simulink model "Controller"  (R2015b)
settings: Solver=FixedStepAuto  StartTime=0.0  StopTime=10.0  FixedStep=0.1  RelTol=1e-3
undefined symbols (not defined in the file): controller_p
libraries: simulink x2
settings Model: Creator=Deepak  LastModifiedBy=Deepak

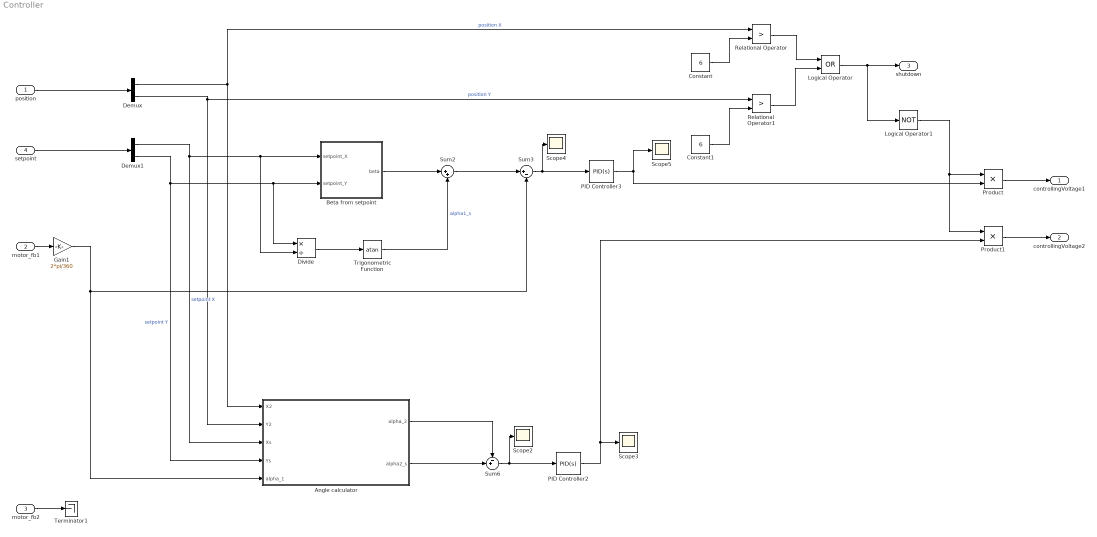
== system Controller ==
  position : Inport
  motor_fb1 : Inport  Port=2
      settings: AttributesFormatString=angle
  motor_fb2 : Inport  Port=3
      settings: AttributesFormatString=angle
  setpoint : Inport  Port=4
      settings: AttributesFormatString=position
  Angle calculator : Subsystem
  Beta from setpoint : Subsystem
  Constant : Constant  Value=6
  Constant1 : Constant  Value=6
  Demux : Demux  Outputs=2
  Demux1 : Demux  Outputs=2
  Divide : Product  Inputs=*/
  Gain1 : Gain  Gain=2*pi/360
  Logical Operator : Logic  Operator=OR  AllPortsSameDT=off  OutDataTypeStr=boolean
  Logical Operator1 : Logic  Operator=NOT  AllPortsSameDT=off  OutDataTypeStr=boolean
  PID Controller2 : simulink/Continuous/PID Controller  Controller=PID  TimeDomain=Continuous-time  SampleTime=-1  IntegratorMethod=Forward Euler  FilterMethod=Forward Euler  Form=Parallel  UseFilter=on  ControllerParametersSource=internal  P=controller_p  I=0  D=0  N=0  InitialConditionSource=internal  InitialConditionForIntegrator=0  InitialConditionForFilter=0  ExternalReset=none  LimitOutput=off  UpperSaturationLimit=inf  LowerSaturationLimit=-inf  LinearizeAsGain=on  AntiWindupMode=none  Kb=1  TrackingMode=off  Kt=1  PParamMin=[]  PParamMax=[]  IParamMin=[]  IParamMax=[]  DParamMin=[]  DParamMax=[]  NParamMin=[]  NParamMax=[]  KbParamMin=[]  KbParamMax=[]  KtParamMin=[]  KtParamMax=[]  POutMin=[]  POutMax=[]  IOutMin=[]  IOutMax=[]  DOutMin=[]  DOutMax=[]  NOutMin=[]  NOutMax=[]  KbOutMin=[]  KbOutMax=[]  KtOutMin=[]  KtOutMax=[]  IntegratorOutMin=[]  IntegratorOutMax=[]  FilterOutMin=[]  FilterOutMax=[]  SumOutMin=[]  SumOutMax=[]  SumI1OutMin=[]  SumI1OutMax=[]  SumI2OutMin=[]  SumI2OutMax=[]  SumI3OutMin=[]  SumI3OutMax=[]  SumDOutMin=[]  SumDOutMax=[]  SaturationOutMin=[]  SaturationOutMax=[]  IntegratorContinuousStateAttributes=''  IntegratorStateMustResolveToSignalObject=off  IntegratorRTWStateStorageClass=Auto  FilterContinuousStateAttributes=''  FilterStateMustResolveToSignalObject=off  FilterRTWStateStorageClass=Auto  DifferentiatorICPrevScaledInput=0  DifferentiatorOutMin=[]  DifferentiatorOutMax=[]
  PID Controller3 : simulink/Continuous/PID Controller  Controller=PID  TimeDomain=Continuous-time  SampleTime=-1  IntegratorMethod=Forward Euler  FilterMethod=Forward Euler  Form=Parallel  UseFilter=on  ControllerParametersSource=internal  P=5/(2*pi)  I=0  D=0  N=0  InitialConditionSource=internal  InitialConditionForIntegrator=0  InitialConditionForFilter=0  ExternalReset=none  LimitOutput=off  UpperSaturationLimit=inf  LowerSaturationLimit=-inf  LinearizeAsGain=on  AntiWindupMode=none  Kb=1  TrackingMode=off  Kt=1  PParamMin=[]  PParamMax=[]  IParamMin=[]  IParamMax=[]  DParamMin=[]  DParamMax=[]  NParamMin=[]  NParamMax=[]  KbParamMin=[]  KbParamMax=[]  KtParamMin=[]  KtParamMax=[]  POutMin=[]  POutMax=[]  IOutMin=[]  IOutMax=[]  DOutMin=[]  DOutMax=[]  NOutMin=[]  NOutMax=[]  KbOutMin=[]  KbOutMax=[]  KtOutMin=[]  KtOutMax=[]  IntegratorOutMin=[]  IntegratorOutMax=[]  FilterOutMin=[]  FilterOutMax=[]  SumOutMin=[]  SumOutMax=[]  SumI1OutMin=[]  SumI1OutMax=[]  SumI2OutMin=[]  SumI2OutMax=[]  SumI3OutMin=[]  SumI3OutMax=[]  SumDOutMin=[]  SumDOutMax=[]  SaturationOutMin=[]  SaturationOutMax=[]  IntegratorContinuousStateAttributes=''  IntegratorStateMustResolveToSignalObject=off  IntegratorRTWStateStorageClass=Auto  FilterContinuousStateAttributes=''  FilterStateMustResolveToSignalObject=off  FilterRTWStateStorageClass=Auto  DifferentiatorICPrevScaledInput=0  DifferentiatorOutMin=[]  DifferentiatorOutMax=[]
  Product : Product
  Product1 : Product
  Relational Operator : RelationalOperator  Operator=>  OutDataTypeStr=boolean
  Relational Operator1 : RelationalOperator  Operator=>  OutDataTypeStr=boolean
  Scope{2..5} (4 alike) : Scope
  Sum2 : Sum  Inputs=|++
  Sum3 : Sum  Inputs=|+-
  Sum6 : Sum  Inputs=-+|
  Terminator1 : Terminator
  Trigonometric Function : Trigonometry  Operator=atan
  controllingVoltage1 : Outport
      settings: AttributesFormatString=voltage
  controllingVoltage2 : Outport  Port=2
      settings: AttributesFormatString=voltage
  shutdown : Outport  Port=3
  wires:
  Constant/1 -> Relational Operator/2
  Constant1/1 -> Relational Operator1/2
  Relational Operator/1 -> Logical Operator/1
  Relational Operator1/1 -> Logical Operator/2
  Logical Operator/1 -> Logical Operator1/1, shutdown/1
  Logical Operator1/1 -> Product1/1, Product/1
  Product/1 -> controllingVoltage1/1
  motor_fb2/1 -> Terminator1/1
  PID Controller2/1 -> Product1/2, Scope3/1
  position/1 -> Demux/1
  setpoint/1 -> Demux1/1
  Sum6/1 -> PID Controller2/1, Scope2/1
  Demux/1 -> Angle calculator/1(X2), Relational Operator/1  "position X"
  Demux/2 -> Relational Operator1/1, Angle calculator/2(Y2)  "position Y"
  Demux1/1 -> Divide/2, Beta from setpoint/1(setpoint_X), Angle calculator/3(Xs)  "setpoint X"
  Demux1/2 -> Angle calculator/4(Ys), Divide/1, Beta from setpoint/2(setpoint_Y)  "setpoint Y"
  Angle calculator/1(alpha_2) -> Sum6/1
  Angle calculator/2(alpha2_s) -> Sum6/2
  Divide/1 -> Trigonometric Function/1
  Trigonometric Function/1 -> Sum2/2  "alpha1_s"
  Beta from setpoint/1(beta) -> Sum2/1
  Sum2/1 -> Sum3/1
  Sum3/1 -> Scope4/1, PID Controller3/1
  PID Controller3/1 -> Product/2, Scope5/1
  Product1/1 -> controllingVoltage2/1
  motor_fb1/1 -> Gain1/1
  Gain1/1 -> Sum3/2, Angle calculator/5(alpha_1)

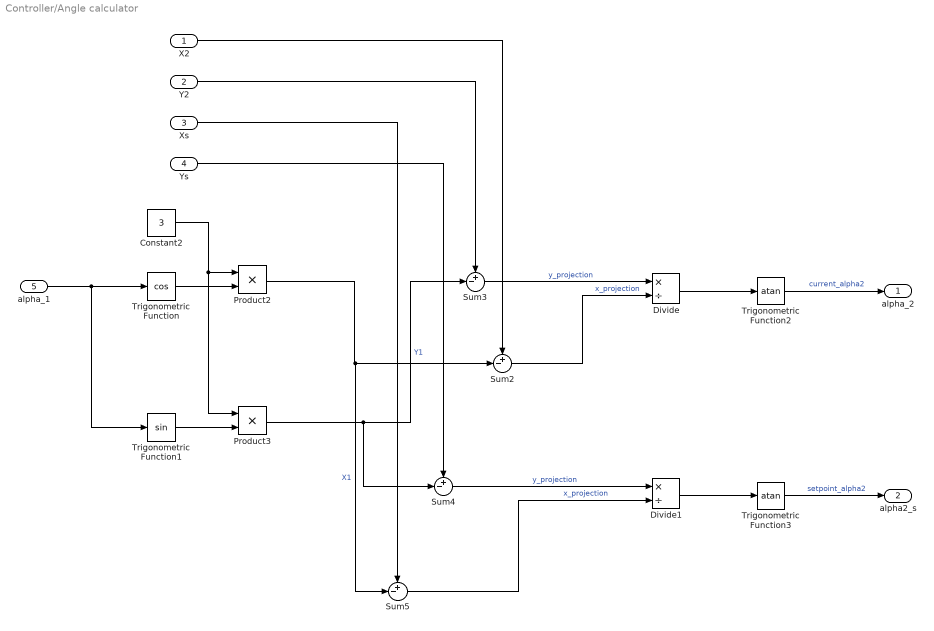
== system Controller/Angle calculator ==
  X2 : Inport
  Y2 : Inport  Port=2
  Xs : Inport  Port=3
  Ys : Inport  Port=4
  alpha_1 : Inport  Port=5
  Constant2 : Constant  Value=3
  Divide : Product  Inputs=*/
  Divide1 : Product  Inputs=*/
  Product2 : Product
  Product3 : Product
  Sum{2..5} (4 alike) : Sum  Inputs=+-|
  Trigonometric Function : Trigonometry  Operator=cos
  Trigonometric Function1 : Trigonometry
  Trigonometric Function2 : Trigonometry  Operator=atan
  Trigonometric Function3 : Trigonometry  Operator=atan
  alpha_2 : Outport
  alpha2_s : Outport  Port=2
  wires:
  X2/1 -> Sum2/1
  Ys/1 -> Sum4/1
  Y2/1 -> Sum3/1
  Xs/1 -> Sum5/1
  Constant2/1 -> Product3/1, Product2/1
  Trigonometric Function/1 -> Product2/2
  Trigonometric Function1/1 -> Product3/2
  alpha_1/1 -> Trigonometric Function1/1, Trigonometric Function/1
  Sum2/1 -> Divide/2  "x_projection"
  Sum3/1 -> Divide/1  "y_projection"
  Product3/1 -> Sum4/2, Sum3/2  "Y1"
  Divide/1 -> Trigonometric Function2/1
  Trigonometric Function2/1 -> alpha_2/1  "current_alpha2"
  Sum5/1 -> Divide1/2  "x_projection"
  Divide1/1 -> Trigonometric Function3/1
  Sum4/1 -> Divide1/1  "y_projection"
  Trigonometric Function3/1 -> alpha2_s/1  "setpoint_alpha2"
  Product2/1 -> Sum5/2, Sum2/2  "X1"

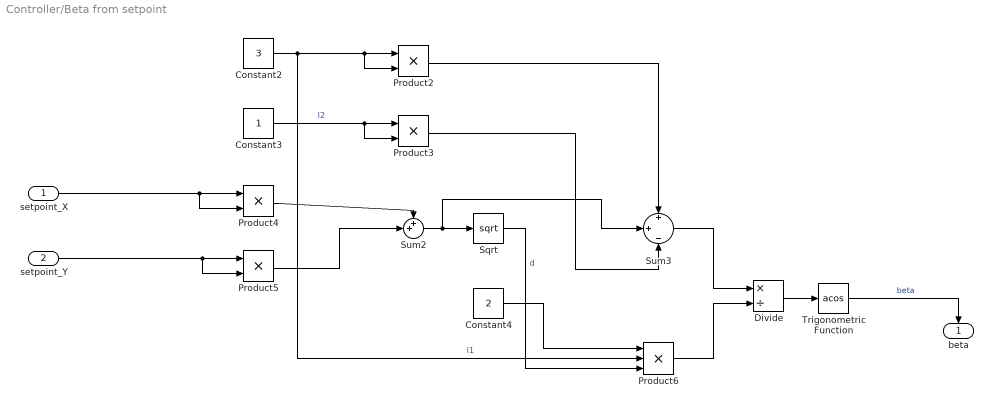
== system Controller/Beta from setpoint ==
  setpoint_X : Inport
  setpoint_Y : Inport  Port=2
  Constant2 : Constant  Value=3
  Constant3 : Constant
  Constant4 : Constant  Value=2
  Divide : Product  Inputs=*/
  Product{2..5} (4 alike) : Product
  Product6 : Product  Inputs=3
  Sqrt : Sqrt  SaturateOnIntegerOverflow=on
  Sum2 : Sum  Inputs=++|
  Sum3 : Sum  Inputs=+|+|-
  Trigonometric Function : Trigonometry  Operator=acos
  beta : Outport
  wires:
  Product2/1 -> Sum3/1
  Product3/1 -> Sum3/3
  Divide/1 -> Trigonometric Function/1
  Product4/1 -> Sum2/1
  Constant2/1 -> Product6/2, Product2/2, Product2/1  "l1"
  Sqrt/1 -> Product6/3  "d"
  Constant3/1 -> Product3/1, Product3/2  "l2"
  Product5/1 -> Sum2/2
  Sum3/1 -> Divide/1
  Constant4/1 -> Product6/1
  setpoint_X/1 -> Product4/2, Product4/1
  setpoint_Y/1 -> Product5/2, Product5/1
  Trigonometric Function/1 -> beta/1  "beta"
  Product6/1 -> Divide/2
  Sum2/1 -> Sum3/2, Sqrt/1
